simulink model "test_cyl_w_hose"  (R2015b)
settings: Solver=ode23t  StartTime=0.0  StopTime=5  FixedStep=1e-6  RelTol=1e-3  AbsTol=1e-4
values from neighbouring files (symbols this model uses):
  a = a_ccfoot * 4.7572e-10    (= 1.522304e-12)    [beta_hose_calc.m]    (also in beta_w_air_entrance.m = 2; param_JOB.m)
  Aa = pi*(Dp^2)/4    (= 0.00020106192983)    [param_JOB.m]
  Ab = pi*(Dp^2-Dr^2)/4    (= 0.00012252211349)    [param_JOB.m]
  Ain = pi*din^2/4    (= 2.82743338823e-05)    [param_JOB.m]
  Aw = 4*V0/DAcc    (= 0.0266666666667)    [param_JOB.m]
  b = b_cc * 3.2808e-6    (= 5.3706696e-07)    [beta_hose_calc.m]    (also in beta_w_air_entrance.m = 1; param_JOB.m)
  beta = 1.4e9    (= 1400000000)    [param_JOB.m]
  beta0 = 1.47e9    (= 1470000000)    [param_JOB.m]
  cf = 0    [param_JOB.m]
  dia = dia_in*2.5e-2    (= 0.0125)    [beta_hose_calc.m]    (also in param_JOB.m = 0.0127)
  fv = 700    [param_JOB.m]
  g1a = 0.004    [param_JOB.m]
  g2a = 0.002    [param_JOB.m]
  h = 10    [param_JOB.m]
  L = 0.5    [beta_hose_calc.m]    (also in param_JOB.m = 0.08)
  leak = 0    [param_JOB.m]
  m_f = 5.6    [param_JOB.m]
  mf = 0    [param_JOB.m]
  Mp = ((pi*Dr^2/4)*L + Aa*0.15)*7860    (= 0.286437851784)    [param_JOB.m]
  n = 1.4    [beta_w_air_entrance.m]    (also in param_JOB.m)
  n2n1 = -1.91    [param_JOB.m]
  nu = nu*1.e-6    (= 3.2e-05)    [param_JOB.m]
  P0 = 100e5    (= 10000000)    [param_JOB.m]
  pAo = ps/2    (= 8000000)    [param_JOB.m]
  pBo = ps/2    (= 8000000)    [param_JOB.m]
  Pmax_acc = 320e5    (= 32000000)    [param_JOB.m]
  pt = 10e5    (= 1000000)    [param_JOB.m]
  Reini = 2500    [param_JOB.m]
  ReT = 2500    [param_JOB.m]
  rho = 800    [param_JOB.m]
  Tamb = 298    [param_JOB.m]
  V0 = A*L    (= 6.13592315154e-05)    [beta_hose_calc.m]    (also in param_JOB.m = 4e-05)
  V0A = v1a + v2a    (= 2.90341084306e-06)    [param_JOB.m]
  V0B = v1b + v2b + v3b    (= 1.67615552692e-06)    [param_JOB.m]
undefined symbols (not defined in the file or in its folder): ah, ah2, bh, bh2, delay, delay2
libraries: simulink x1
settings Model: Creator=Toshiba  LastModifiedBy=Toshiba

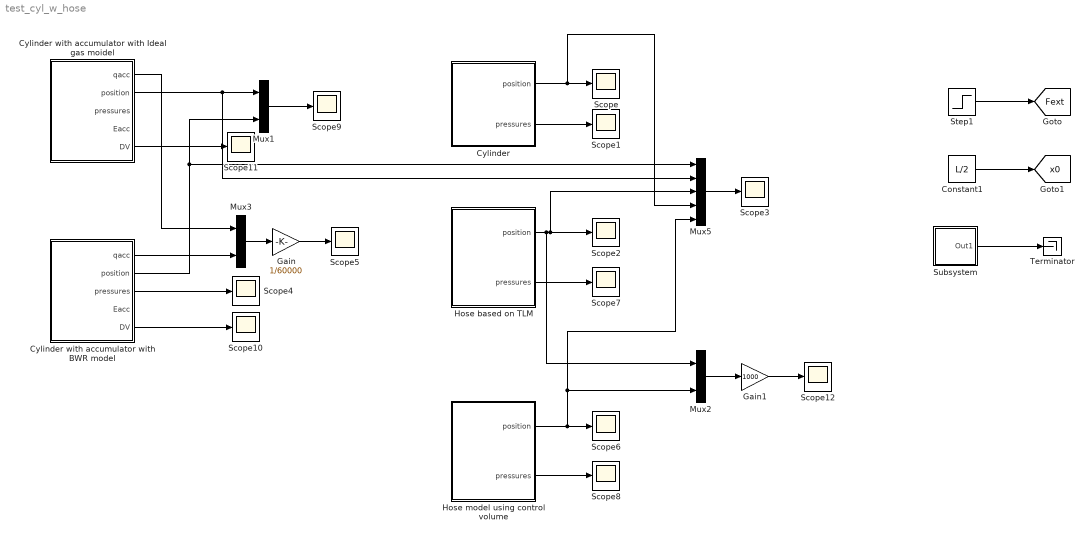
== system test_cyl_w_hose ==
  Constant1 : Constant  Value=L/2
  Cylinder : Subsystem
  Cylinder with accumulator with BWR model : Subsystem
  Cylinder with accumulator with Ideal gas moidel : Subsystem
  Gain : Gain  Gain=1/60000
  Gain1 : Gain  Gain=1000
  Hose based on TLM : Subsystem
  "Hose model using control volume " : Subsystem
  Mux1 : Mux  Inputs=2
  Mux2 : Mux  Inputs=2
  Mux3 : Mux  Inputs=2
  Mux5 : Mux  Inputs=5
  Scope{,1..12} (13 alike) : Scope
  Step1 : Step  Time=2  After=500  SampleTime=0
  Subsystem : Subsystem
  Terminator : Terminator
  tag scope: Fext=global, x0=global
  wires:
  Step1/1 -> [Fext]
  Constant1/1 -> [x0]
  Cylinder/1(position) -> Mux5/4, Scope/1
  Hose based on TLM/1(position) -> Mux2/1, Mux5/3, Scope2/1
  Hose based on TLM/2(pressures) -> Scope7/1
  Cylinder with accumulator with Ideal gas moidel/2(position) -> Mux5/2, Mux1/1
  Cylinder/2(pressures) -> Scope1/1
  Cylinder with accumulator with BWR model/2(position) -> Mux1/2, Mux5/1
  Mux1/1 -> Scope9/1
  Subsystem/1(Out1) -> Terminator/1
  Mux5/1 -> Scope3/1
  Mux3/1 -> Gain/1
  Gain/1 -> Scope5/1
  Cylinder with accumulator with BWR model/3(pressures) -> Scope4/1
  Cylinder with accumulator with BWR model/1(qacc) -> Mux3/2
  Cylinder with accumulator with Ideal gas moidel/1(qacc) -> Mux3/1
  "Hose model using control volume "/1(position) -> Mux5/5, Mux2/2, Scope6/1
  "Hose model using control volume "/2(pressures) -> Scope8/1
  Cylinder with accumulator with BWR model/5(DV) -> Scope10/1
  Cylinder with accumulator with Ideal gas moidel/5(DV) -> Scope11/1
  Mux2/1 -> Gain1/1
  Gain1/1 -> Scope12/1

== system test_cyl_w_hose/Cylinder ==
  Constant : Constant  Value=0
  Cylinder HOERBIGER LB6 1610 0080 4M1 : Subsystem
  Mux : Mux  Inputs=2
  Subsystem : Subsystem
  position : Outport
  pressures : Outport  Port=2
  wires:
  Cylinder HOERBIGER LB6 1610 0080 4M1/2(pA) -> Mux/1
  Cylinder HOERBIGER LB6 1610 0080 4M1/3(pB) -> Subsystem/1(In1)
  Mux/1 -> pressures/1
  Cylinder HOERBIGER LB6 1610 0080 4M1/1(xA) -> position/1
  [Fext] -> Cylinder HOERBIGER LB6 1610 0080 4M1/3(Fext)
  [x0] -> Cylinder HOERBIGER LB6 1610 0080 4M1/4(xLo)
  Constant/1 -> Cylinder HOERBIGER LB6 1610 0080 4M1/2(qB), Cylinder HOERBIGER LB6 1610 0080 4M1/1(qA)
  Subsystem/1(Out1) -> Mux/2

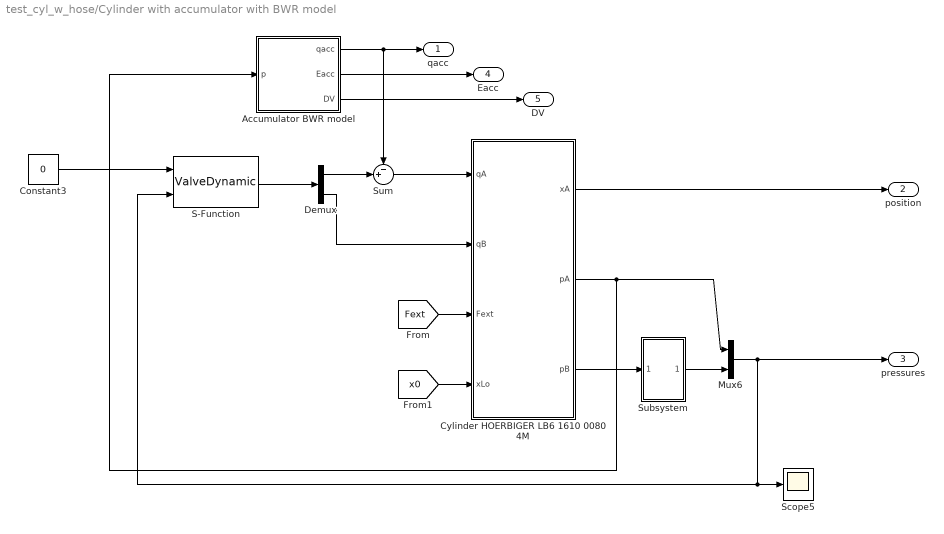
== system test_cyl_w_hose/Cylinder with accumulator with BWR model ==
  Accumulator BWR model : Subsystem
  Constant3 : Constant  Value=0
  Cylinder HOERBIGER LB6 1610 0080 4M : Subsystem
  Demux : Demux  Outputs=2
  Mux6 : Mux  Inputs=2
  S-Function : S-Function  FunctionName=ValveDynamic  Parameters=wn, E, In, Kva, Kvb, KvlkA, KvlkB, ps, pt,up_dz,lw_dz  SFunctionDeploymentMode=off  EnableBusSupport=off
  Scope5 : Scope
  Subsystem : Subsystem
  Sum : Sum  Inputs=-+|
  qacc : Outport
  position : Outport  Port=2
  pressures : Outport  Port=3
  Eacc : Outport  Port=4
  DV : Outport  Port=5
  wires:
  Sum/1 -> Cylinder HOERBIGER LB6 1610 0080 4M/1(qA)
  Mux6/1 -> S-Function/2, Scope5/1, pressures/1
  Cylinder HOERBIGER LB6 1610 0080 4M/2(pA) -> Accumulator BWR model/1(p), Mux6/1
  Cylinder HOERBIGER LB6 1610 0080 4M/1(xA) -> position/1
  [x0] -> Cylinder HOERBIGER LB6 1610 0080 4M/4(xLo)
  [Fext] -> Cylinder HOERBIGER LB6 1610 0080 4M/3(Fext)
  Accumulator BWR model/2(Eacc) -> Eacc/1
  Accumulator BWR model/1(qacc) -> qacc/1, Sum/1
  Constant3/1 -> S-Function/1
  S-Function/1 -> Demux/1
  Demux/1 -> Sum/2
  Demux/2 -> Cylinder HOERBIGER LB6 1610 0080 4M/2(qB)
  Accumulator BWR model/3(DV) -> DV/1
  Cylinder HOERBIGER LB6 1610 0080 4M/3(pB) -> Subsystem/1(In1)
  Subsystem/1(Out1) -> Mux6/2

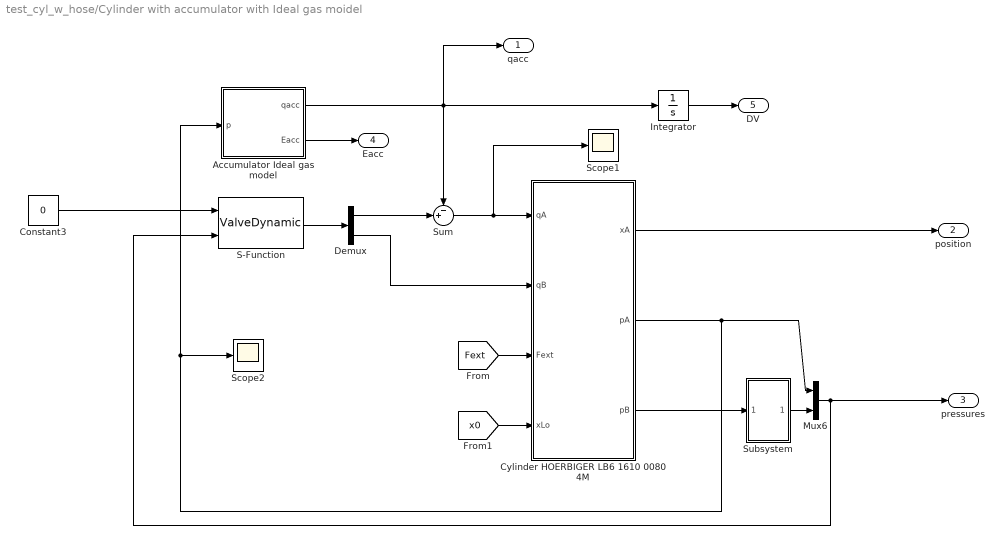
== system test_cyl_w_hose/Cylinder with accumulator with Ideal gas moidel ==
  Accumulator Ideal gas model : Subsystem
  Constant3 : Constant  Value=0
  Cylinder HOERBIGER LB6 1610 0080 4M : Subsystem
  Demux : Demux  Outputs=2
  Integrator : Integrator
  Mux6 : Mux  Inputs=2
  S-Function : S-Function  FunctionName=ValveDynamic  Parameters=wn, E, In, Kva, Kvb, KvlkA, KvlkB, ps, pt,up_dz,lw_dz  SFunctionDeploymentMode=off  EnableBusSupport=off
  Scope1 : Scope
  Scope2 : Scope
  Subsystem : Subsystem
  Sum : Sum  Inputs=-+|
  qacc : Outport
  position : Outport  Port=2
  pressures : Outport  Port=3
  Eacc : Outport  Port=4
  DV : Outport  Port=5
  wires:
  [Fext] -> Cylinder HOERBIGER LB6 1610 0080 4M/3(Fext)
  [x0] -> Cylinder HOERBIGER LB6 1610 0080 4M/4(xLo)
  Cylinder HOERBIGER LB6 1610 0080 4M/3(pB) -> Subsystem/1(In1)
  Cylinder HOERBIGER LB6 1610 0080 4M/1(xA) -> position/1
  Cylinder HOERBIGER LB6 1610 0080 4M/2(pA) -> Accumulator Ideal gas model/1(p), Scope2/1, Mux6/1
  Mux6/1 -> S-Function/2, pressures/1
  Demux/1 -> Sum/2
  Accumulator Ideal gas model/1(qacc) -> qacc/1, Integrator/1, Sum/1
  Sum/1 -> Scope1/1, Cylinder HOERBIGER LB6 1610 0080 4M/1(qA)
  Accumulator Ideal gas model/2(Eacc) -> Eacc/1
  Constant3/1 -> S-Function/1
  S-Function/1 -> Demux/1
  Demux/2 -> Cylinder HOERBIGER LB6 1610 0080 4M/2(qB)
  Integrator/1 -> DV/1
  Subsystem/1(Out1) -> Mux6/2

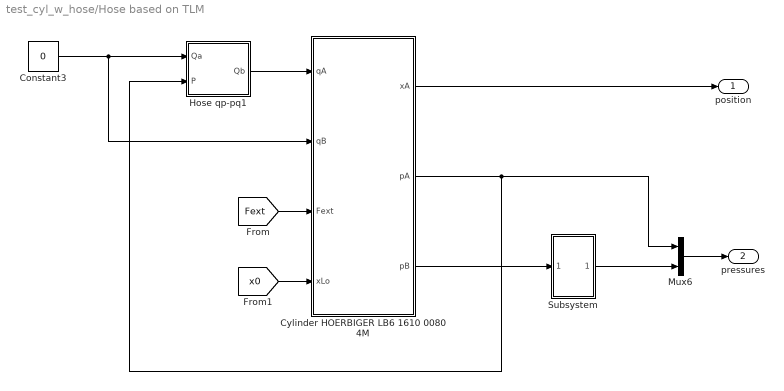
== system test_cyl_w_hose/Hose based on TLM ==
  Constant3 : Constant  Value=0
  Cylinder HOERBIGER LB6 1610 0080 4M : Subsystem
  Hose qp-pq1 : Subsystem
  Mux6 : Mux  Inputs=2
  Subsystem : Subsystem
  position : Outport
  pressures : Outport  Port=2
  wires:
  Constant3/1 -> Cylinder HOERBIGER LB6 1610 0080 4M/2(qB), Hose qp-pq1/1(Qa)
  Mux6/1 -> pressures/1
  Cylinder HOERBIGER LB6 1610 0080 4M/2(pA) -> Hose qp-pq1/2(P), Mux6/1
  Cylinder HOERBIGER LB6 1610 0080 4M/1(xA) -> position/1
  Cylinder HOERBIGER LB6 1610 0080 4M/3(pB) -> Subsystem/1(In1)
  [x0] -> Cylinder HOERBIGER LB6 1610 0080 4M/4(xLo)
  [Fext] -> Cylinder HOERBIGER LB6 1610 0080 4M/3(Fext)
  Hose qp-pq1/1(Qb) -> Cylinder HOERBIGER LB6 1610 0080 4M/1(qA)
  Subsystem/1(Out1) -> Mux6/2

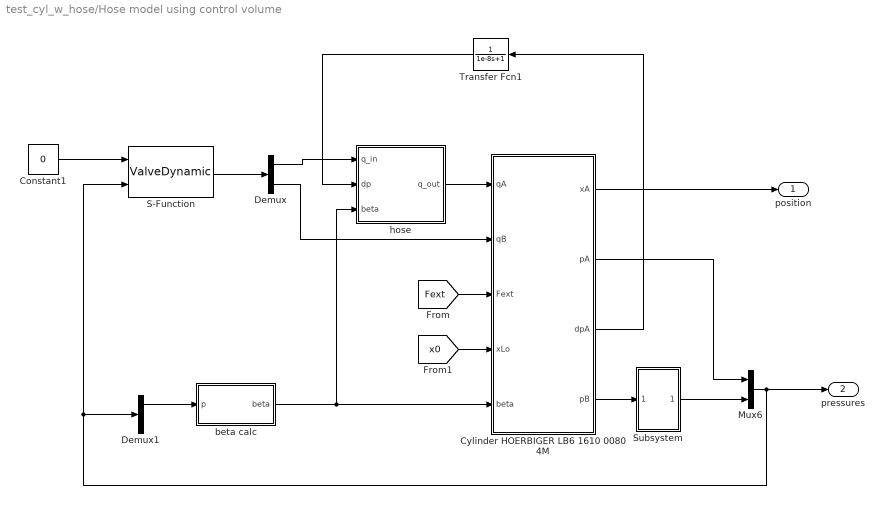
== system test_cyl_w_hose/Hose model using control volume  ==
  Constant1 : Constant  Value=0
  Cylinder HOERBIGER LB6 1610 0080 4M : Subsystem
  Demux : Demux  Outputs=2
  Demux1 : Demux  Outputs=2
  Mux6 : Mux  Inputs=2
  S-Function : S-Function  FunctionName=ValveDynamic  Parameters=wn, E, In, Kva, Kvb, KvlkA, KvlkB, ps, pt,up_dz,lw_dz  SFunctionDeploymentMode=off  EnableBusSupport=off
  Subsystem : Subsystem
  Transfer Fcn1 : TransferFcn  Denominator=[1e-8 1]
  beta calc : MATLAB Function  TreatAsAtomicUnit=on
  hose : MATLAB Function  TreatAsAtomicUnit=on
  position : Outport
  pressures : Outport  Port=2
  wires:
  hose/1(q_out) -> Cylinder HOERBIGER LB6 1610 0080 4M/1(qA)
  [Fext] -> Cylinder HOERBIGER LB6 1610 0080 4M/3(Fext)
  [x0] -> Cylinder HOERBIGER LB6 1610 0080 4M/4(xLo)
  Cylinder HOERBIGER LB6 1610 0080 4M/1(xA) -> position/1
  Cylinder HOERBIGER LB6 1610 0080 4M/2(pA) -> Mux6/1
  Mux6/1 -> S-Function/2, Demux1/1, pressures/1
  Constant1/1 -> S-Function/1
  Demux/1 -> hose/1(q_in)
  Demux/2 -> Cylinder HOERBIGER LB6 1610 0080 4M/2(qB)
  Cylinder HOERBIGER LB6 1610 0080 4M/4(pB) -> Subsystem/1(In1)
  Subsystem/1(Out1) -> Mux6/2
  beta calc/1(beta) -> hose/3(beta), Cylinder HOERBIGER LB6 1610 0080 4M/5(beta)
  Demux1/1 -> beta calc/1(p)
  Cylinder HOERBIGER LB6 1610 0080 4M/3(dpA) -> Transfer Fcn1/1
  Transfer Fcn1/1 -> hose/2(dp)
  S-Function/1 -> Demux/1

== system test_cyl_w_hose/Subsystem ==
  Ramp1 : simulink/Sources/Ramp  slope=800  start=2  X0=0
  Saturation1 : Saturate  UpperLimit=50000  LowerLimit=0
  Out1 : Outport
  wires:
  Saturation1/1 -> Out1/1
  Ramp1/1 -> Saturation1/1

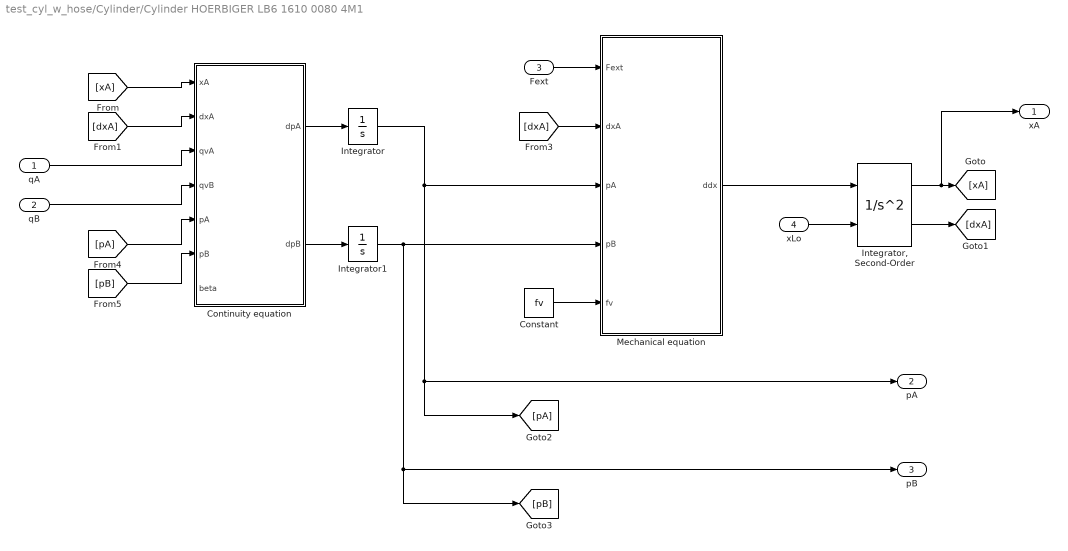
== system test_cyl_w_hose/Cylinder/Cylinder HOERBIGER LB6 1610 0080 4M1 ==
  qA : Inport
  qB : Inport  Port=2
  Fext : Inport  Port=3
  xLo : Inport  Port=4
  Constant : Constant  Value=fv
  Continuity equation : MATLAB Function  TreatAsAtomicUnit=on
  Integrator : Integrator  InitialCondition=pAo
  "Integrator, Second-Order" : SecondOrderIntegrator  ICSourceX=external  ICX=xo  LimitX=on  UpperLimitX=L  LowerLimitX=0
  Integrator1 : Integrator  InitialCondition=pBo
  Mechanical equation : MATLAB Function  TreatAsAtomicUnit=on
  xA : Outport
  pA : Outport  Port=2
  pB : Outport  Port=3
  wires:
  Continuity equation/1(dpA) -> Integrator/1
  Continuity equation/2(dpB) -> Integrator1/1
  Integrator/1 -> Mechanical equation/3(pA), [pA], pA/1
  Integrator1/1 -> pB/1, [pB], Mechanical equation/4(pB)
  qA/1 -> Continuity equation/3(qvA)
  qB/1 -> Continuity equation/4(qvB)
  Mechanical equation/1(ddx) -> "Integrator, Second-Order"/1
  [dxA] -> Continuity equation/2(dxA)
  [xA] -> Continuity equation/1(xA)
  "Integrator, Second-Order"/1 -> xA/1, [xA]
  "Integrator, Second-Order"/2 -> [dxA]
  Constant/1 -> Mechanical equation/5(fv)
  [dxA] -> Mechanical equation/2(dxA)
  [pA] -> Continuity equation/5(pA)
  [pB] -> Continuity equation/6(pB)
  Fext/1 -> Mechanical equation/1(Fext)
  xLo/1 -> "Integrator, Second-Order"/2

== system test_cyl_w_hose/Cylinder/Subsystem ==
  In1 : Inport
  Constant1 : Constant  Value=pt
  Gain : Gain  Gain=0
  Sum1 : Sum  Inputs=|++
  Out1 : Outport
  wires:
  Sum1/1 -> Out1/1
  Constant1/1 -> Sum1/2
  In1/1 -> Gain/1
  Gain/1 -> Sum1/1

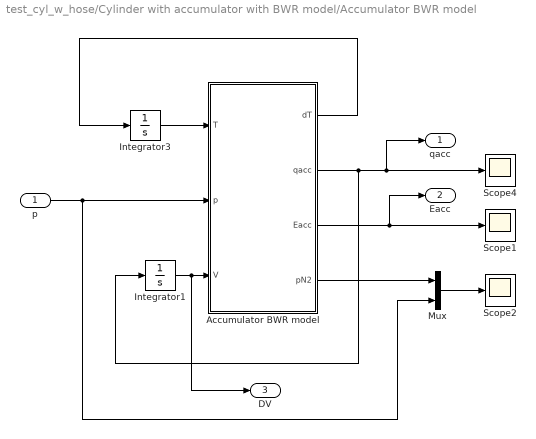
== system test_cyl_w_hose/Cylinder with accumulator with BWR model/Accumulator BWR model ==
  p : Inport
  Accumulator BWR model : MATLAB Function  TreatAsAtomicUnit=on
  Integrator1 : Integrator  UpperSaturationLimit=V0  LowerSaturationLimit=0
  Integrator3 : Integrator  InitialCondition=Tamb  LowerSaturationLimit=0
  Mux : Mux  Inputs=2
  Scope1 : Scope
  Scope2 : Scope
  Scope4 : Scope
  qacc : Outport
  Eacc : Outport  Port=2
  DV : Outport  Port=3
  wires:
  p/1 -> Accumulator BWR model/2(p), Mux/2
  Accumulator BWR model/1(dT) -> Integrator3/1
  Mux/1 -> Scope2/1
  Integrator3/1 -> Accumulator BWR model/1(T)
  Accumulator BWR model/2(qacc) -> Integrator1/1, qacc/1, Scope4/1
  Integrator1/1 -> DV/1, Accumulator BWR model/3(V)
  Accumulator BWR model/3(Eacc) -> Eacc/1, Scope1/1
  Accumulator BWR model/4(pN2) -> Mux/1

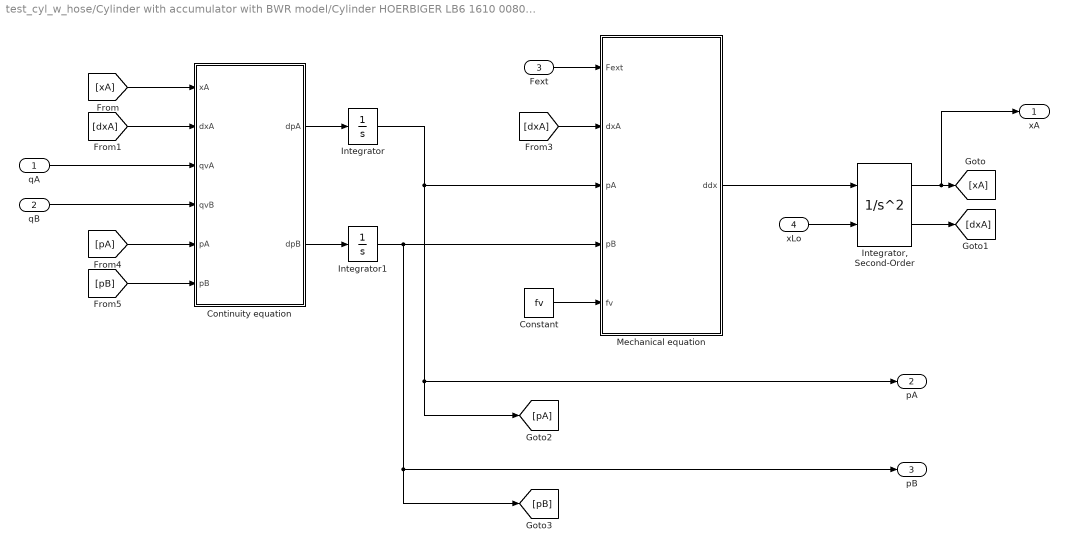
== system test_cyl_w_hose/Cylinder with accumulator with BWR model/Cylinder HOERBIGER LB6 1610 0080 4M ==
  qA : Inport
  qB : Inport  Port=2
  Fext : Inport  Port=3
  xLo : Inport  Port=4
  Constant : Constant  Value=fv
  Continuity equation : MATLAB Function  TreatAsAtomicUnit=on
  Integrator : Integrator  InitialCondition=pAo
  "Integrator, Second-Order" : SecondOrderIntegrator  ICSourceX=external  ICX=xo  LimitX=on  UpperLimitX=L  LowerLimitX=0
  Integrator1 : Integrator  InitialCondition=pBo
  Mechanical equation : MATLAB Function  TreatAsAtomicUnit=on
  xA : Outport
  pA : Outport  Port=2
  pB : Outport  Port=3
  wires:
  xLo/1 -> "Integrator, Second-Order"/2
  Fext/1 -> Mechanical equation/1(Fext)
  [pB] -> Continuity equation/6(pB)
  [pA] -> Continuity equation/5(pA)
  [dxA] -> Mechanical equation/2(dxA)
  Constant/1 -> Mechanical equation/5(fv)
  "Integrator, Second-Order"/2 -> [dxA]
  "Integrator, Second-Order"/1 -> [xA], xA/1
  [xA] -> Continuity equation/1(xA)
  [dxA] -> Continuity equation/2(dxA)
  Mechanical equation/1(ddx) -> "Integrator, Second-Order"/1
  qB/1 -> Continuity equation/4(qvB)
  qA/1 -> Continuity equation/3(qvA)
  Integrator1/1 -> Mechanical equation/4(pB), [pB], pB/1
  Integrator/1 -> pA/1, [pA], Mechanical equation/3(pA)
  Continuity equation/2(dpB) -> Integrator1/1
  Continuity equation/1(dpA) -> Integrator/1

== system test_cyl_w_hose/Cylinder with accumulator with BWR model/Subsystem ==
  In1 : Inport
  Constant1 : Constant  Value=pt
  Gain : Gain  Gain=0
  Sum1 : Sum  Inputs=|++
  Out1 : Outport
  wires:
  Gain/1 -> Sum1/1
  In1/1 -> Gain/1
  Constant1/1 -> Sum1/2
  Sum1/1 -> Out1/1

== system test_cyl_w_hose/Cylinder with accumulator with Ideal gas moidel/Accumulator Ideal gas model ==
  p : Inport
  Accumulator ideal gas model : MATLAB Function  TreatAsAtomicUnit=on
  Integrator1 : Integrator  InitialCondition=P0  LimitOutput=on  UpperSaturationLimit=Pmax_acc  LowerSaturationLimit=P0
  qacc : Outport
  Eacc : Outport  Port=2
  wires:
  Integrator1/1 -> Accumulator ideal gas model/2(pacc)
  Accumulator ideal gas model/2(dp) -> Integrator1/1
  Accumulator ideal gas model/1(qacc) -> qacc/1
  p/1 -> Accumulator ideal gas model/1(p)
  Accumulator ideal gas model/3(Eacc) -> Eacc/1

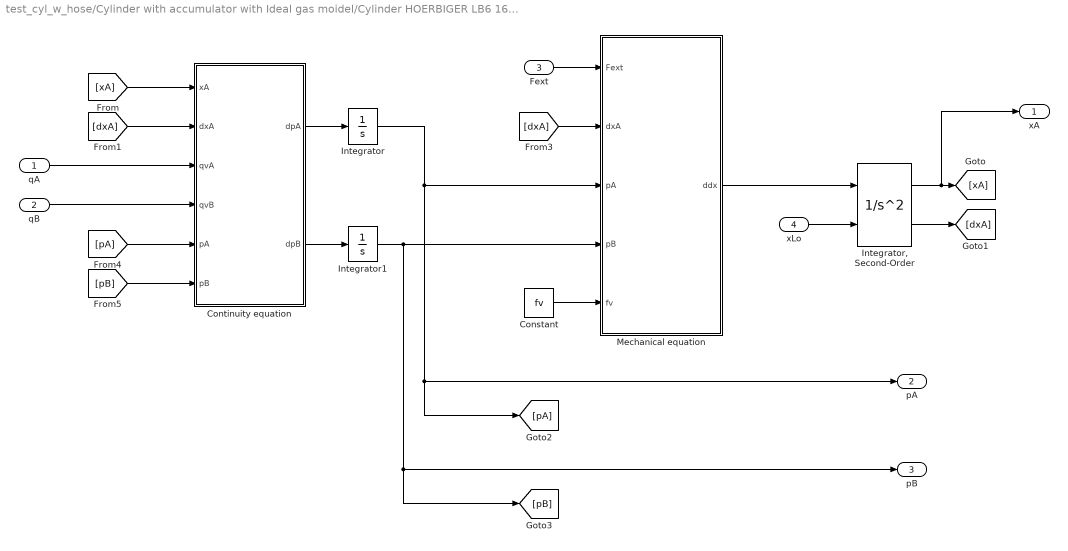
== system test_cyl_w_hose/Cylinder with accumulator with Ideal gas moidel/Cylinder HOERBIGER LB6 1610 0080 4M ==
  qA : Inport
  qB : Inport  Port=2
  Fext : Inport  Port=3
  xLo : Inport  Port=4
  Constant : Constant  Value=fv
  Continuity equation : MATLAB Function  TreatAsAtomicUnit=on
  Integrator : Integrator  InitialCondition=pAo
  "Integrator, Second-Order" : SecondOrderIntegrator  ICSourceX=external  ICX=xo  LimitX=on  UpperLimitX=L  LowerLimitX=0
  Integrator1 : Integrator  InitialCondition=pBo
  Mechanical equation : MATLAB Function  TreatAsAtomicUnit=on
  xA : Outport
  pA : Outport  Port=2
  pB : Outport  Port=3
  wires:
  Continuity equation/1(dpA) -> Integrator/1
  Continuity equation/2(dpB) -> Integrator1/1
  Integrator/1 -> Mechanical equation/3(pA), [pA], pA/1
  Integrator1/1 -> pB/1, [pB], Mechanical equation/4(pB)
  qA/1 -> Continuity equation/3(qvA)
  qB/1 -> Continuity equation/4(qvB)
  Mechanical equation/1(ddx) -> "Integrator, Second-Order"/1
  [dxA] -> Continuity equation/2(dxA)
  [xA] -> Continuity equation/1(xA)
  "Integrator, Second-Order"/1 -> xA/1, [xA]
  "Integrator, Second-Order"/2 -> [dxA]
  Constant/1 -> Mechanical equation/5(fv)
  [dxA] -> Mechanical equation/2(dxA)
  [pA] -> Continuity equation/5(pA)
  [pB] -> Continuity equation/6(pB)
  Fext/1 -> Mechanical equation/1(Fext)
  xLo/1 -> "Integrator, Second-Order"/2

== system test_cyl_w_hose/Cylinder with accumulator with Ideal gas moidel/Subsystem ==
  In1 : Inport
  Constant1 : Constant  Value=pt
  Gain : Gain  Gain=0
  Sum1 : Sum  Inputs=|++
  Out1 : Outport
  wires:
  Gain/1 -> Sum1/1
  In1/1 -> Gain/1
  Constant1/1 -> Sum1/2
  Sum1/1 -> Out1/1

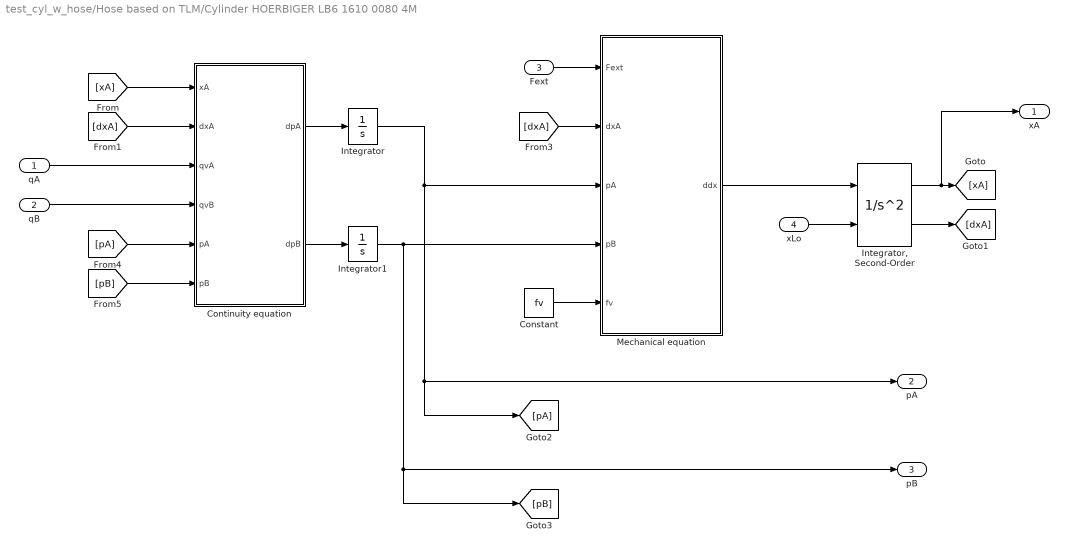
== system test_cyl_w_hose/Hose based on TLM/Cylinder HOERBIGER LB6 1610 0080 4M ==
  qA : Inport
  qB : Inport  Port=2
  Fext : Inport  Port=3
  xLo : Inport  Port=4
  Constant : Constant  Value=fv
  Continuity equation : MATLAB Function  TreatAsAtomicUnit=on
  Integrator : Integrator  InitialCondition=pAo
  "Integrator, Second-Order" : SecondOrderIntegrator  ICSourceX=external  ICX=xo  LimitX=on  UpperLimitX=L  LowerLimitX=0
  Integrator1 : Integrator  InitialCondition=pBo
  Mechanical equation : MATLAB Function  TreatAsAtomicUnit=on
  xA : Outport
  pA : Outport  Port=2
  pB : Outport  Port=3
  wires:
  xLo/1 -> "Integrator, Second-Order"/2
  Fext/1 -> Mechanical equation/1(Fext)
  [pB] -> Continuity equation/6(pB)
  [pA] -> Continuity equation/5(pA)
  [dxA] -> Mechanical equation/2(dxA)
  Constant/1 -> Mechanical equation/5(fv)
  "Integrator, Second-Order"/2 -> [dxA]
  "Integrator, Second-Order"/1 -> [xA], xA/1
  [xA] -> Continuity equation/1(xA)
  [dxA] -> Continuity equation/2(dxA)
  Mechanical equation/1(ddx) -> "Integrator, Second-Order"/1
  qB/1 -> Continuity equation/4(qvB)
  qA/1 -> Continuity equation/3(qvA)
  Integrator1/1 -> Mechanical equation/4(pB), [pB], pB/1
  Integrator/1 -> pA/1, [pA], Mechanical equation/3(pA)
  Continuity equation/2(dpB) -> Integrator1/1
  Continuity equation/1(dpA) -> Integrator/1

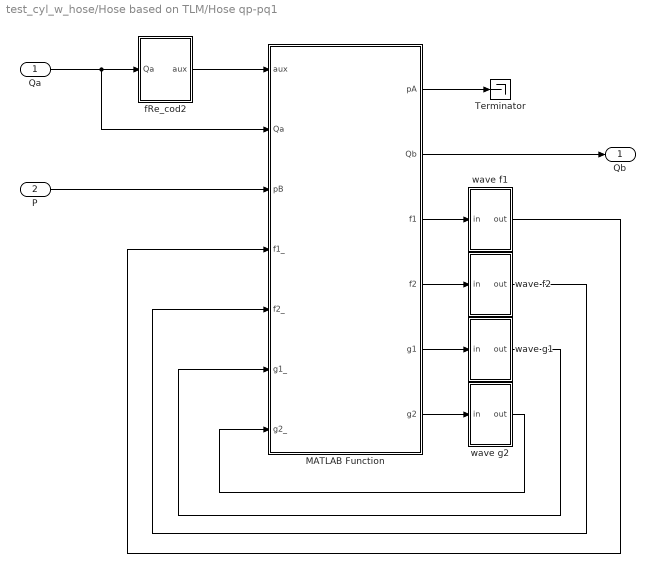
== system test_cyl_w_hose/Hose based on TLM/Hose qp-pq1 ==
  Qa : Inport
  P : Inport  Port=2
  MATLAB Function : MATLAB Function  TreatAsAtomicUnit=on
  Terminator : Terminator
  fRe_cod2 : Subsystem
  wave f1 : Subsystem
  wave f2 : Subsystem
  wave g1 : Subsystem
  wave g2 : Subsystem
  Qb : Outport
  wires:
  fRe_cod2/1(aux) -> MATLAB Function/1(aux)
  Qa/1 -> MATLAB Function/2(Qa), fRe_cod2/1(Qa)
  MATLAB Function/3(f1) -> wave f1/1(in)
  MATLAB Function/4(f2) -> wave f2/1(in)
  MATLAB Function/5(g1) -> wave g1/1(in)
  MATLAB Function/6(g2) -> wave g2/1(in)
  MATLAB Function/2(Qb) -> Qb/1
  MATLAB Function/1(pA) -> Terminator/1
  P/1 -> MATLAB Function/3(pB)
  wave f1/1(out) -> MATLAB Function/4(f1_)
  wave f2/1(out) -> MATLAB Function/5(f2_)
  wave g1/1(out) -> MATLAB Function/6(g1_)
  wave g2/1(out) -> MATLAB Function/7(g2_)

== system test_cyl_w_hose/Hose based on TLM/Subsystem ==
  In1 : Inport
  Constant1 : Constant  Value=pt
  Gain : Gain  Gain=0
  Sum1 : Sum  Inputs=|++
  Out1 : Outport
  wires:
  Gain/1 -> Sum1/1
  In1/1 -> Gain/1
  Constant1/1 -> Sum1/2
  Sum1/1 -> Out1/1

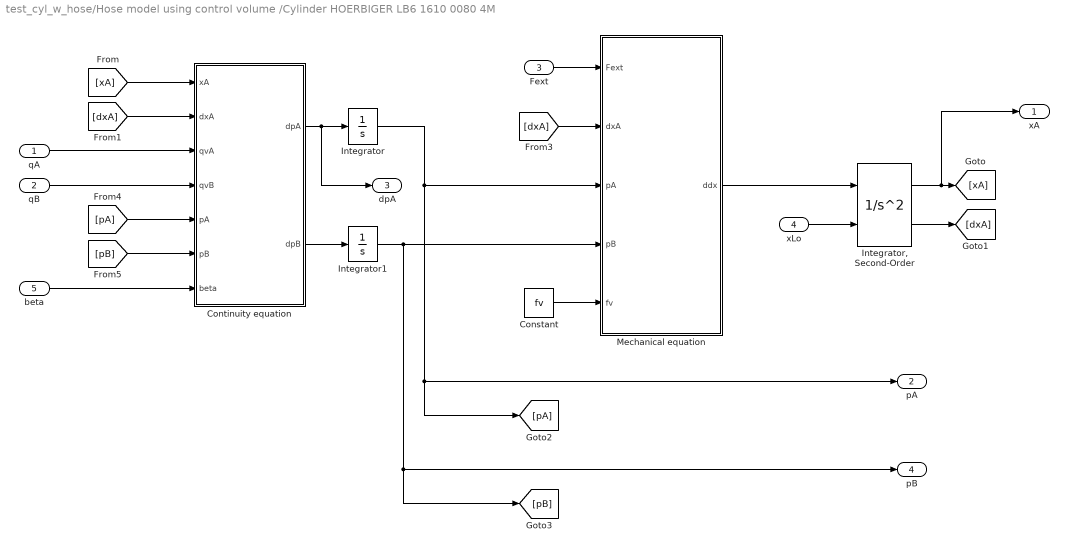
== system test_cyl_w_hose/Hose model using control volume /Cylinder HOERBIGER LB6 1610 0080 4M ==
  qA : Inport
  qB : Inport  Port=2
  Fext : Inport  Port=3
  xLo : Inport  Port=4
  beta : Inport  Port=5
  Constant : Constant  Value=fv
  Continuity equation : MATLAB Function  TreatAsAtomicUnit=on
  Integrator : Integrator  InitialCondition=pAo
  "Integrator, Second-Order" : SecondOrderIntegrator  ICSourceX=external  ICX=xo  LimitX=on  UpperLimitX=L  LowerLimitX=0
  Integrator1 : Integrator  InitialCondition=pBo
  Mechanical equation : MATLAB Function  TreatAsAtomicUnit=on
  xA : Outport
  pA : Outport  Port=2
  dpA : Outport  Port=3
  pB : Outport  Port=4
  wires:
  Continuity equation/1(dpA) -> dpA/1, Integrator/1
  Continuity equation/2(dpB) -> Integrator1/1
  Integrator/1 -> Mechanical equation/3(pA), [pA], pA/1
  Integrator1/1 -> pB/1, [pB], Mechanical equation/4(pB)
  qA/1 -> Continuity equation/3(qvA)
  qB/1 -> Continuity equation/4(qvB)
  Mechanical equation/1(ddx) -> "Integrator, Second-Order"/1
  [dxA] -> Continuity equation/2(dxA)
  [xA] -> Continuity equation/1(xA)
  "Integrator, Second-Order"/1 -> xA/1, [xA]
  "Integrator, Second-Order"/2 -> [dxA]
  Constant/1 -> Mechanical equation/5(fv)
  [dxA] -> Mechanical equation/2(dxA)
  [pA] -> Continuity equation/5(pA)
  [pB] -> Continuity equation/6(pB)
  Fext/1 -> Mechanical equation/1(Fext)
  xLo/1 -> "Integrator, Second-Order"/2
  beta/1 -> Continuity equation/7(beta)

== system test_cyl_w_hose/Hose model using control volume /Subsystem ==
  In1 : Inport
  Constant1 : Constant  Value=pt
  Gain : Gain  Gain=0
  Sum1 : Sum  Inputs=|++
  Out1 : Outport
  wires:
  Sum1/1 -> Out1/1
  Constant1/1 -> Sum1/2
  In1/1 -> Gain/1
  Gain/1 -> Sum1/1

== system test_cyl_w_hose/Hose based on TLM/Hose qp-pq1/fRe_cod2 ==
  Qa : Inport
  Integrator1 : Integrator  InitialCondition=0.042
  Integrator2 : Integrator  InitialCondition=Reini  LimitOutput=on  LowerSaturationLimit=ReT
  MATLAB Function : MATLAB Function  TreatAsAtomicUnit=on
  MATLAB Function2 : MATLAB Function  TreatAsAtomicUnit=on
  aux : Outport
  wires:
  Integrator2/1 -> MATLAB Function/1(Re_), MATLAB Function2/1(Re_)
  Qa/1 -> MATLAB Function/3(Qa), MATLAB Function2/3(Qa)
  MATLAB Function2/1(dRe_) -> Integrator2/1
  Integrator1/1 -> MATLAB Function/2(aux)
  MATLAB Function/3(daux) -> Integrator1/1
  MATLAB Function/1(out) -> aux/1
  MATLAB Function/2(fRe) -> MATLAB Function2/2(fRe)

== system test_cyl_w_hose/Hose based on TLM/Hose qp-pq1/wave f1 ==
  in : Inport
  Constant : Constant  Value=ah
  Constant1 : Constant  Value=bh
  Integrator1 : Integrator
  MATLAB Function : MATLAB Function  TreatAsAtomicUnit=on
  Transport Delay : TransportDelay  DelayTime=delay
  out : Outport
  wires:
  Constant1/1 -> MATLAB Function/3(b)
  Constant/1 -> MATLAB Function/2(a)
  Transport Delay/1 -> out/1
  in/1 -> MATLAB Function/1(u)
  MATLAB Function/1(daux) -> Integrator1/1
  Integrator1/1 -> MATLAB Function/4(aux)
  MATLAB Function/2(S) -> Transport Delay/1

== system test_cyl_w_hose/Hose based on TLM/Hose qp-pq1/wave f2 ==
  in : Inport
  Constant : Constant  Value=ah2
  Constant1 : Constant  Value=bh2
  Integrator1 : Integrator
  MATLAB Function : MATLAB Function  TreatAsAtomicUnit=on
  Transport Delay : TransportDelay  DelayTime=delay2
  out : Outport
  wires:
  MATLAB Function/2(S) -> Transport Delay/1
  Integrator1/1 -> MATLAB Function/4(aux)
  MATLAB Function/1(daux) -> Integrator1/1
  in/1 -> MATLAB Function/1(u)
  Transport Delay/1 -> out/1
  Constant/1 -> MATLAB Function/2(a)
  Constant1/1 -> MATLAB Function/3(b)

== system test_cyl_w_hose/Hose based on TLM/Hose qp-pq1/wave g1 ==
  in : Inport
  Constant : Constant  Value=ah
  Constant1 : Constant  Value=bh
  Integrator1 : Integrator
  MATLAB Function : MATLAB Function  TreatAsAtomicUnit=on
  Transport Delay : TransportDelay  DelayTime=delay
  out : Outport
  wires:
  MATLAB Function/2(S) -> Transport Delay/1
  Integrator1/1 -> MATLAB Function/4(aux)
  MATLAB Function/1(daux) -> Integrator1/1
  in/1 -> MATLAB Function/1(u)
  Transport Delay/1 -> out/1
  Constant/1 -> MATLAB Function/2(a)
  Constant1/1 -> MATLAB Function/3(b)

== system test_cyl_w_hose/Hose based on TLM/Hose qp-pq1/wave g2 ==
  in : Inport
  Constant : Constant  Value=ah2
  Constant1 : Constant  Value=bh2
  Integrator1 : Integrator
  MATLAB Function : MATLAB Function  TreatAsAtomicUnit=on
  Transport Delay : TransportDelay  DelayTime=delay2
  out : Outport
  wires:
  Constant1/1 -> MATLAB Function/3(b)
  Constant/1 -> MATLAB Function/2(a)
  Transport Delay/1 -> out/1
  in/1 -> MATLAB Function/1(u)
  MATLAB Function/1(daux) -> Integrator1/1
  Integrator1/1 -> MATLAB Function/4(aux)
  MATLAB Function/2(S) -> Transport Delay/1

== matlab function test_cyl_w_hose/Hose based on TLM/Cylinder HOERBIGER LB6 1610 0080 4M/Continuity equation ==
  data: xA input; dpA output; dpB output; dxA input; qvA input; qvB input; pA input; pB input; leak parameter; V0A parameter; V0B parameter; Aa parameter; Ab parameter; L parameter; beta parameter
function [dpA,dpB] = fcn(xA, dxA, qvA, qvB, pA, pB, leak, V0A, V0B, Aa, Ab, L, beta)

pC = pA - pB;   % Pressao de carga [Pa]

qvlk = leak * pC;
     
dpa = (beta/(V0A + Aa*xA)) * (qvA - Aa*dxA - qvlk);
dpb = (beta/(V0B + Ab*(L-xA))) * (Ab*dxA + qvlk - qvB);

dpA = dpa;
dpB = dpb;

== matlab function test_cyl_w_hose/Hose based on TLM/Cylinder HOERBIGER LB6 1610 0080 4M/Mechanical equation ==
  data: Fext input; dxA input; ddx output; pA input; pB input; fv input; Aa parameter; Ab parameter; Mp parameter
function ddx = fcn(Fext, dxA, pA, pB, fv, Aa, Ab, Mp)
%#codegen

FH  = pA*Aa - pB*Ab;                % N - Hydraulic force
Ffr = fv*dxA;                       % N - Friction force (Viscous)

ddx = (FH - Ffr - Fext)/Mp;        % m/s2 - Acceleration

== matlab function test_cyl_w_hose/Cylinder/Cylinder HOERBIGER LB6 1610 0080 4M1/Continuity equation ==
  data: xA input; dpA output; dpB output; dxA input; qvA input; qvB input; pA input; pB input; leak parameter; V0A parameter; V0B parameter; Aa parameter; Ab parameter; L parameter; beta input
function [dpA,dpB] = fcn(xA, dxA, qvA, qvB, pA, pB, leak, V0A, V0B, Aa, Ab, L, beta)

pC = pA - pB;   % Pressao de carga [Pa]

qvlk = leak * pC;
     
dpa = (beta/(V0A + Aa*xA)) * (qvA - Aa*dxA - qvlk);
dpb = (beta/(V0B + Ab*(L-xA))) * (Ab*dxA + qvlk - qvB);

dpA = dpa;
dpB = dpb;

== matlab function test_cyl_w_hose/Hose based on TLM/Hose qp-pq1/wave g1/MATLAB Function ==
  data: u input; daux output; a input; b input; aux input; S output
function [daux,S] = fcn(u,a,b,aux)
%#codegen

daux = a.*u - b.*aux;
S = sum(aux);

== matlab function test_cyl_w_hose/Hose based on TLM/Hose qp-pq1/wave f2/MATLAB Function ==
  data: u input; daux output; a input; b input; aux input; S output
function [daux,S] = fcn(u,a,b,aux)
%#codegen

daux = a.*u - b.*aux;
S = sum(aux);

== matlab function test_cyl_w_hose/Cylinder/Cylinder HOERBIGER LB6 1610 0080 4M1/Mechanical equation ==
  data: Fext input; dxA input; ddx output; pA input; pB input; fv input; Aa parameter; Ab parameter; Mp parameter
function ddx = fcn(Fext, dxA, pA, pB, fv, Aa, Ab, Mp)
%#codegen

FH  = pA*Aa - pB*Ab;                % N - Hydraulic force
Ffr = fv*dxA;                       % N - Friction force (Viscous)

ddx = (FH - Ffr - Fext)/Mp;        % m/s2 - Acceleration

== matlab function test_cyl_w_hose/Cylinder with accumulator with Ideal gas moidel/Cylinder HOERBIGER LB6 1610 0080 4M/Continuity equation ==
  data: xA input; dpA output; dpB output; dxA input; qvA input; qvB input; pA input; pB input; leak parameter; V0A parameter; V0B parameter; Aa parameter; Ab parameter; L parameter; beta parameter
function [dpA,dpB] = fcn(xA, dxA, qvA, qvB, pA, pB, leak, V0A, V0B, Aa, Ab, L, beta)

pC = pA - pB;   % Pressao de carga [Pa]

qvlk = leak * pC;
     
dpa = (beta/(V0A + Aa*xA)) * (qvA - Aa*dxA - qvlk);
dpb = (beta/(V0B + Ab*(L-xA))) * (Ab*dxA + qvlk - qvB);

dpA = dpa;
dpB = dpb;

== matlab function test_cyl_w_hose/Cylinder with accumulator with Ideal gas moidel/Cylinder HOERBIGER LB6 1610 0080 4M/Mechanical equation ==
  data: Fext input; dxA input; ddx output; pA input; pB input; fv input; Aa parameter; Ab parameter; Mp parameter
function ddx = fcn(Fext, dxA, pA, pB, fv, Aa, Ab, Mp)
%#codegen

FH  = pA*Aa - pB*Ab;                % N - Hydraulic force
Ffr = fv*dxA;                       % N - Friction force (Viscous)

ddx = (FH - Ffr - Fext)/Mp;        % m/s2 - Acceleration

== matlab function test_cyl_w_hose/Cylinder with accumulator with BWR model/Accumulator BWR model/Accumulator BWR model ==
  data: T input; p input; V input; dT output; Tamb parameter; h parameter; Aw parameter; P0 parameter; Pmax_acc parameter; V0 parameter; mf parameter; cf parameter; qacc output; Ain parameter; rho parameter; Eacc output; pN2 output
% ====================================================
% Code made by 
% JOB A. LEDEZMA, 2016
% ....................
% Special thanks to RAFAEL BRAVO from LASHIP/UFSC
% for his help in this matter.
% ====================================================

% The dynamic modeling of the accumulator is based on the following 
% references:

% POURMOVAHED, A., BEACHLEY, N. H.,FRONCZAK, F. J. 
% "Modeling of a Hydraulic Energy Regeneration System - Part I: Analytical Treatment"
% Journal of Dynamic Systems, Measurement, and Control, 1992, ASME
% ....................................................................
% ECHTER, Nicholas
% "Parallel hydraulic pressure assist/work circuit hybrids for Automated side loader refuse vehicles"
% Master Thesis, Department of Mechanical Engineering, Colorado State University
% United States, 2012
% ....................................................................


function [dT,qacc,Eacc,pN2] = fcn(T,p,V,Tamb,h,Aw,P0,Pmax_acc,V0,mf,cf,Ain,rho)
%#codegen

% DATA OF CONSTANTS VALUES
% ========================
% Ao,a,Bo,b,Co,c,alpha,gamma  :  constants in BWR equation
Ao = 136.0436;      % (m^3/Kg)^2·Pa
Bo = 1.454397e-3;   % m^3/Kg
Co = 1040558;       % (m^3/Kg)^2·K^2·Pa
a = 1.156984e-1;    % (m^3/Kg)^3·Pa
b = 2.966165e-6;    % (m^3/Kg)^2
c = 3357.338;       % (m^3/Kg)^3·K^2·Pa
alpha = 5.786149e-9;% (m^3/Kg)^3
gamma = 6.753738e-6;% (m^3/Kg)^2

R = 296.7923;       % m^3·Pa/(Kg·K) : gas constant
Cd = 0.67;          % Discharge coefficient

N1 = -735.210;      % K^3
N2 = 34.224;        % K^2
N3 = -0.557648;     % K
N4 = 3.5040;        
N5 = -1.7339e-5;    % K^-1
N6 = 1.7465e-8;     % K^-2
N7 = -3.5689e-12;   % K^-3
N8 = 1.0054;        
N9 = 3353.4061;     % K

KN2 = 1.04;         % Compressibility factor of the nitrogen under load condition of the accumulator

% Mass of the internal gas
mg  = P0*V0/(R*Tamb*KN2);% Kg

% Gas specific volume
if V >= V0
    V = V0;
else if V < 0
        V = 0;
    end
end
Vl = V;
v = (V0 - V)/mg;    % m^3/Kg

% Gas Pressure = f(gas temperature, specific volume)
% Benedict-Webb-Rubin (BWR) equation of state

pg = R*T/v + (Bo*R*T - Ao - Co/T^2)/v^2 + (b*R*T - a)/v^3 +...
    a*alpha/v^6 + c*(1 + gamma/v^2)*exp(-gamma/v^2)/(v^3*T^2);  % Pa

if pg <= P0
    pN2 = P0;
else if pg >= Pmax_acc
        pN2 = Pmax_acc;
    else
        pN2 = pg;
    end
end

% Volumetric flow rate
if (p<P0)
    qacc = 0;
else
    qacc = sign(p - pN2)*Cd*Ain*sqrt(2*abs(p-pN2)/rho);
end    

% Constant-volume specific heat of gas
cv = (N1/T^3 + N2/T^2 + N3/T + (N4-1) + N5*T + N6*T^2 + N7*T^3 + ...
     N8*(N9/T)^2*((exp(N9/T))/(exp(N9/T) - 1)^2))*R + ...
     (6/T^3)*(Co/v - c/gamma) + (3*c/T^3)*(2/gamma + 1/v^2)*...
     exp(-gamma/v^2); % J/(Kg·K)

% Accumulator thermal time constant
tau = mg *cv / (h*Aw); % s

% Specific volume rate
dv = -(qacc/mg);   % m^3/(s·Kg)

% 1st derivative of the absolute gas or foam temperature
dT = (((Tamb - T)/tau) - (dv/cv)*((R*T/v)*(1 + b/v^2) + ...
    (1/v^2)*(Bo*R*T + 2*Co/T^2) - (2*c/(v^3*T^2))*(1 + gamma/v^2) * ...
    exp(-gamma/v^2))) / (1 + mf*cf/(mg*cv)); % K/s

% Storage energy
Eacc = (pN2-P0)*v*mg;
% Eacc = (V0*P0^(1/n))*(pN2^((n-1)/n) - P0^((n-1)/n))/(n-1);

== matlab function test_cyl_w_hose/Cylinder with accumulator with Ideal gas moidel/Accumulator Ideal gas model/Accumulator ideal gas model ==
  data: qacc output; p input; pacc input; dp output; V0 parameter; P0 parameter; n parameter; Ain parameter; rho parameter; Eacc output
function [qacc,dp,Eacc] = fcn(p,pacc,V0,P0,n,Ain,rho)
% function q = fcn(p,dp)
%#codegen

Cd = 0.67;

% Flow rate through a restriction
if (p<P0) && (pacc <= P0)
    qacc = 0;
else
    qacc = sign(p - pacc)*Cd*Ain*sqrt(2*abs(p-pacc)/rho);
end    

% Accumulator capacitance
Cacc = (V0*P0^(1/n))/(n* (p+1e5)^((n+1)/n));
% V = 

% Pressure rate
dp =  Cacc^-1 * qacc;

% Stored energy 
Eacc = (V0*P0^(1/n))*(p^((n-1)/n) - P0^((n-1)/n))/(n-1);

== matlab function test_cyl_w_hose/Hose based on TLM/Hose qp-pq1/wave f1/MATLAB Function ==
  data: u input; daux output; a input; b input; aux input; S output
function [daux,S] = fcn(u,a,b,aux)
%#codegen

daux = a.*u - b.*aux;
S = sum(aux);

== matlab function test_cyl_w_hose/Hose based on TLM/Hose qp-pq1/wave g2/MATLAB Function ==
  data: u input; daux output; a input; b input; aux input; S output
function [daux,S] = fcn(u,a,b,aux)
%#codegen

daux = a.*u - b.*aux;
S = sum(aux);

== matlab function test_cyl_w_hose/Cylinder with accumulator with BWR model/Cylinder HOERBIGER LB6 1610 0080 4M/Continuity equation ==
  data: xA input; dpA output; dpB output; dxA input; qvA input; qvB input; pA input; pB input; leak parameter; V0A parameter; V0B parameter; Aa parameter; Ab parameter; L parameter; beta parameter
function [dpA,dpB] = fcn(xA, dxA, qvA, qvB, pA, pB, leak, V0A, V0B, Aa, Ab, L, beta)

pC = pA - pB;   % Pressao de carga [Pa]

qvlk = leak * pC;
     
dpa = (beta/(V0A + Aa*xA)) * (qvA - Aa*dxA - qvlk);
dpb = (beta/(V0B + Ab*(L-xA))) * (Ab*dxA + qvlk - qvB);

dpA = dpa;
dpB = dpb;

== matlab function test_cyl_w_hose/Cylinder with accumulator with BWR model/Cylinder HOERBIGER LB6 1610 0080 4M/Mechanical equation ==
  data: Fext input; dxA input; ddx output; pA input; pB input; fv input; Aa parameter; Ab parameter; Mp parameter
function ddx = fcn(Fext, dxA, pA, pB, fv, Aa, Ab, Mp)
%#codegen

FH  = pA*Aa - pB*Ab;                % N - Hydraulic force
Ffr = fv*dxA;                       % N - Friction force (Viscous)

ddx = (FH - Ffr - Fext)/Mp;        % m/s2 - Acceleration

== matlab function test_cyl_w_hose/Hose based on TLM/Hose qp-pq1/MATLAB Function ==
  data: aux input; pA output; Qa input; pB input; f1_ input; f2_ input; g1_ input; g2_ input; rho parameter; g1a parameter; g2a parameter; dia parameter; n2n1 parameter; Qb output; f1 output; f2 output; g1 output; g2 output
% ====================================================
% Code made by 
% JOB A. LEDEZMA, 2016
% ..............................
% The present model is a translation of model 
% proposed by Prof. D. N. Johnston 
% University of Bath - England
% the original simulink block model can be downloaded from:
% http://people.bath.ac.uk/ensdnj/models/hose.html
% ====================================================

% The dynamic modeling of the hose is based on the following reference:
 
% JOHNSTON, D. N. 
% "A time-domain model of axial wave propagation in 
%  liquid-filled flexible hoses"
%  Proc IMechE, part I, Vol 220, No. 7, pp. 517-530
% ....................................................................

function [pA,Qb,f1,f2,g1,g2] = fcn(aux,Qa,pB,f1_,f2_,g1_,g2_,rho,g1a,g2a,dia,n2n1)
%#codegen

area = pi*dia^2/4;              % m2 - hose section
n1n2 = 1 / n2n1;                % ratio of modal ratios

% Speed of waves
c1 = 1/g1a;
c2 = 1/g2a;
% Characteristic impedances
Z1 = rho*c1*(1.5-exp(-(pB*1e-5)/50));                   
Z2 = rho*c2*(1.5-exp(-(pB*1e-5)/50));
% Forward traveling waves equations
f1 = Qa/(area*(1-n1n2)) - g1_;
f2 = Qa/(area*(1-n2n1)) - g2_;
% Backward traveling waves equations
g1 = (f1_*(Z1 + n1n2 * Z2) + f2_*2*Z2 - pB) * (1/(Z1 - n1n2 * Z2));
g2 = (f1_*2*Z1 + f2_*(Z2 + n2n1 * Z1) - pB) * (1/(Z2 - n2n1 * Z1));

% Flowrate at port B
Qb = area*(f1_ + f2_ + g1 + g2);
% Pressure at port A
pA = aux + Z1*(f1 - g1_)+ Z2*(f2 - g2_);

== matlab function test_cyl_w_hose/Hose model using control volume /Cylinder HOERBIGER LB6 1610 0080 4M/Continuity equation ==
  data: xA input; dpA output; dpB output; dxA input; qvA input; qvB input; pA input; pB input; leak parameter; V0A parameter; V0B parameter; Aa parameter; Ab parameter; L parameter; beta input
function [dpA,dpB] = fcn(xA, dxA, qvA, qvB, pA, pB, leak, V0A, V0B, Aa, Ab, L, beta)

pC = pA - pB;   % Pressao de carga [Pa]

qvlk = leak * pC;
     
dpA = (beta/(V0A + Aa*xA)) * (qvA - Aa*dxA - qvlk);
dpB = (beta/(V0B + Ab*(L-xA))) * (Ab*dxA + qvlk - qvB);

== matlab function test_cyl_w_hose/Hose based on TLM/Hose qp-pq1/fRe_cod2/MATLAB Function ==
  data: Re_ input; out output; fRe output; aux input; daux output; ReT parameter; nu parameter; rho parameter; length parameter; dia parameter; Qa input
function [out,fRe,daux] = fcn(Re_,aux,ReT,nu,rho,length,dia,Qa)
%#codegen

if Re_>ReT
    fRe = 0.25*Re_*(2*log10(Re_*sqrt(aux)) - 0.8)^-2;
else fRe = 16;
end
daux = 100*((2*log10(Re_*sqrt(aux)) - 0.8)^-2 - aux);
out = Qa* fRe * (8*nu*rho*length/(pi*dia^4));

== matlab function test_cyl_w_hose/Hose based on TLM/Hose qp-pq1/fRe_cod2/MATLAB Function2 ==
  data: Re_ input; fRe input; dRe_ output; Qa input; dia parameter; nu parameter
function dRe_ = fcn(Re_,fRe,Qa,dia,nu)
%#codegen

Re = abs(Qa)*4/(pi*dia*nu);
Re_sat = Re;
if Re <= 2500
    Re_sat = 2500;
end
H = log(sign(Re_*fRe*0.5)*sqrt(abs(Re_*fRe*0.5))) + 2.2;
tauB = (1/H * (1-1.5/H) * (1-2/H))*(250*dia^2/nu)/ Re_sat;
dRe_ = (Re - Re_)/tauB;

== matlab function test_cyl_w_hose/Hose model using control volume /Cylinder HOERBIGER LB6 1610 0080 4M/Mechanical equation ==
  data: Fext input; dxA input; ddx output; pA input; pB input; fv input; Aa parameter; Ab parameter; Mp parameter
function ddx = fcn(Fext, dxA, pA, pB, fv, Aa, Ab, Mp)
%#codegen

FH  = pA*Aa - pB*Ab;                % N - Hydraulic force
Ffr = fv*dxA;                       % N - Friction force (Viscous)

ddx = (FH - Ffr - Fext)/Mp;        % m/s2 - Acceleration

== matlab function test_cyl_w_hose/Hose model using control volume /hose ==
  data: q_in input; dp input; beta input; q_out output; length parameter; dia parameter; a parameter
function q_out = fcn(q_in,dp,beta,length,dia,a)
%#codegen

Ah = pi*dia^2/4;
V0h = Ah*length;

q_out = q_in - (a*length - V0h/beta)*dp;

== matlab function test_cyl_w_hose/Hose model using control volume /beta calc ==
  data: p input; m_f parameter; beta0 parameter; beta output; dia parameter; a parameter; b parameter
function beta = fcn(p,m_f,beta0,dia,a,b)
%#codegen


% fluid bulk modulus
beta_f = beta0 + m_f*p;   % Pa - Secant definition
% beta_f = beta0 + (1+(m_f - 1)*p/beta0)*(1 + m_f*p/beta0);   % Pa - tangent definition

% hose bulk modulus
Ah = pi*dia^2/4; 
% V0h = Ah*length;
bbias = (Ah + b)/a;
beta_hose = p + bbias;

% effective bulk modulus
beta = beta_f * beta_hose / (beta_f + beta_hose);
